simulink model "Lista4"  (R2023a)
settings: Solver=VariableStepAuto  StartTime=0.0  StopTime=10.0  RelTol=1e-3
libraries: fl_lib x8, nesl_utility x3
settings Model: Creator=gutoc  LastModifiedBy=gutoc

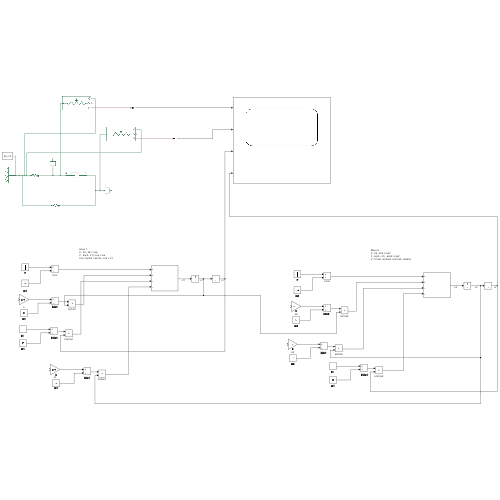
[thumbnail: Simulink's stored preview of the top-level diagram]
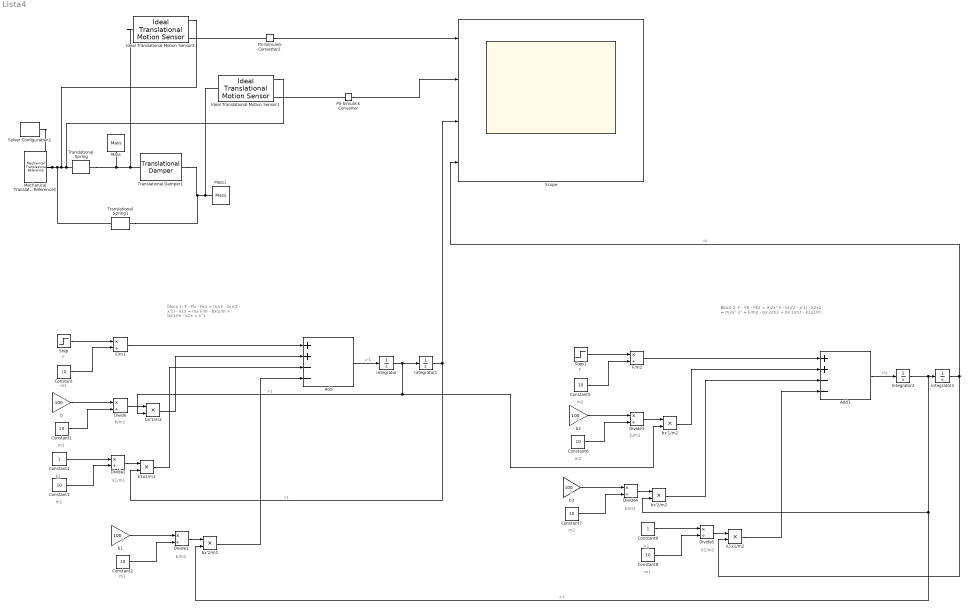
== system Lista4 ==
  note: Bloco 2:
      | F - Fb - Fk2 = m2x''
      | F - b(x'2 - x'1) - k2x2 = m2x"
      | x" = F/m2 - bx'2/m2 + bx'1/m2 - k2x2/m
  note: b
  note: m2
  note: b/m1
  note: m1
  note: k1
  note: m2
  note: k1/m1
  note: b/m2
  note: F
  note: m2
  note: b
  note: b
  note: bloco 1:
      | F - Fb - Fk1 = ma
      | F - b(x'2 - x'1) - k1x = ma
      | F/m - bx'2/m + bx'1/m - k1x = x"1
  note: m1
  note: m1
  note: b/m1
  note: m1
  note: k1
  note: m1
  note: k1/m1
  note: b/m1
  note: F
  Add : Sum  Inputs=++--
  Add1 : Sum  Inputs=++--
  Constant{,1..3,5..8} (8 alike) : Constant  Value=10
  Constant4 : Constant
  Constant9 : Constant
  Divide{,1..5} (6 alike) : Product  Inputs=*/
  F/m1 : Product  Inputs=*/
  F/m2 : Product  Inputs=*/
  Ideal Translational Motion Sensor1 : fl_lib/Mechanical/Mechanical Sensors/Ideal Translational Motion Sensor  reference=foundation.enum.MeasurementReference.difference  acceleration_port=false  velocity_port=true  position_port=true  offset=0 m
  Ideal Translational Motion Sensor3 : fl_lib/Mechanical/Mechanical Sensors/Ideal Translational Motion Sensor  reference=foundation.enum.MeasurementReference.difference  acceleration_port=false  velocity_port=true  position_port=true  offset=0 m
  Integrator{,1..3} (4 alike) : Integrator
  Mass : fl_lib/Mechanical/Translational Elements/Mass  mass=1 kg  num_ports=foundation.enum.numPorts2.one  v_specify=off  v_priority=High  v=0 m/s  v_nominal_specify=off  v_nominal_unit=m/s  v_nominal_value=1  f_specify=off  f_priority=None  f=0 N  f_nominal_specify=off  f_nominal_unit=N  f_nominal_value=1
  Mass1 : fl_lib/Mechanical/Translational Elements/Mass  mass=2 kg  num_ports=foundation.enum.numPorts2.one  v_specify=off  v_priority=High  v=0 m/s  v_nominal_specify=off  v_nominal_unit=m/s  v_nominal_value=1  f_specify=off  f_priority=None  f=0 N  f_nominal_specify=off  f_nominal_unit=N  f_nominal_value=1
  Mechanical Translational Reference1 : fl_lib/Mechanical/Translational Elements/Mechanical Translational Reference
  PS-Simulink Converter : nesl_utility/PS-Simulink Converter  PhysicalDomain=network_engine_domain  SubClassName=ps_output  LeftPortType=input  RightPortType=output  PseudoPeriodic=off  Frequencies=[]  VectorFormat=inherit  Unit=inherit  AffineConversion=off
  PS-Simulink Converter2 : nesl_utility/PS-Simulink Converter  PhysicalDomain=network_engine_domain  SubClassName=ps_output  LeftPortType=input  RightPortType=output  PseudoPeriodic=off  Frequencies=[]  VectorFormat=inherit  Unit=inherit  AffineConversion=off
  Scope : Scope  NumInputPorts=4
  Solver Configuration1 : nesl_utility/Solver Configuration  PhysicalDomain=network_engine_domain  SubClassName=solver  LeftPortType=input  RightPortType=generic  Tones=[]  Harmonics=[]  SimulateNoise=off  Profile=off  UseLocalSampling=off  EnableSwitchedLinearOptims=on  FrequencyDomain=off  UseCCode=off  RelTol=0.001  AbsTol=1e-06  MinStep=1e-09  ToWorkspace=off  RevertToSquareIcSolve=off  NumHomotopyIterations=100  PhasorMode=off  PhasorModeNumHarmonics=1  ConsistencySolver=NEWTON_FTOL  IndexReductionMethod=DerivativeReplacement  DoDC=off  ResidualTolerance=1e-09  ConsistencyTolSource=GLOBAL  ConsistencyAbsTol=0.001  ConsistencyRelTol=0.001  ConsistencyTolFactor=0.001  UseLocalSolver=off  LocalSolverChoice=NE_BACKWARD_EULER_ADVANCER  ResolveIndetEquations=on  FunctionEvalNumThread=1  LocalSolverSampleTime=0.001  DoFixedCost=off  MaxNonlinIter=3  MaxModeIter=2  ComputeImpulses=off  ImpulseIterations=2  LinearAlgebra=Sparse  LinearAlgebraNumThread=0  EquationFormulation=NE_TIME_EF  DelaysMemoryBudget=1024  AutomaticFiltering=on  FilteringTimeConstant=0.001  PartitionStorageMethod=AS_NEEDED  PartitionMemoryBudget=1024  PartitionMethod=FAST
  Step : Step  SampleTime=0
  Step1 : Step  SampleTime=0
  Translational Damper1 : fl_lib/Mechanical/Translational Elements/Translational Damper  D=100 N/(m/s)  v_specify=off  v_priority=None  v=0 m/s  v_nominal_specify=off  v_nominal_unit=m/s  v_nominal_value=1  f_specify=off  f_priority=None  f=0 N  f_nominal_specify=off  f_nominal_unit=N  f_nominal_value=1
  Translational Spring : fl_lib/Mechanical/Translational Elements/Translational Spring  spr_rate=1000 N/m  v_specify=off  v_priority=None  v=0 m/s  v_nominal_specify=off  v_nominal_unit=m/s  v_nominal_value=1  f_specify=off  f_priority=None  f=0 N  f_nominal_specify=off  f_nominal_unit=N  f_nominal_value=1  x_specify=off  x_priority=High  x=0 m  x_nominal_specify=off  x_nominal_unit=m  x_nominal_value=1
  Translational Spring1 : fl_lib/Mechanical/Translational Elements/Translational Spring  spr_rate=1000 N/m  v_specify=off  v_priority=None  v=0 m/s  v_nominal_specify=off  v_nominal_unit=m/s  v_nominal_value=1  f_specify=off  f_priority=None  f=0 N  f_nominal_specify=off  f_nominal_unit=N  f_nominal_value=1  x_specify=off  x_priority=High  x=0 m  x_nominal_specify=off  x_nominal_unit=m  x_nominal_value=1
  b{,1..3} (4 alike) : Gain  Gain=100
  bx'1/m1 : Product
  bx'1/m2 : Product
  bx'2/m1 : Product
  bx'2/m2 : Product
  k1x1/m1 : Product
  k1x1/m2 : Product
  wires:
  PS-Simulink Converter/1 -> Scope/2
  PS-Simulink Converter2/1 -> Scope/1
  bx'2/m2/1 -> Add1/3
  F/m2/1 -> Add1/1
  Step1/1 -> F/m2/1
  Divide4/1 -> bx'2/m2/1
  b3/1 -> Divide4/1
  Constant7/1 -> Divide4/2
  Divide3/1 -> bx'1/m2/1
  Constant9/1 -> Divide5/1
  Constant6/1 -> Divide3/2
  Divide5/1 -> k1x1/m2/1
  Constant8/1 -> Divide5/2
  Integrator2/1 -> bx'2/m1/2, bx'2/m2/2, Integrator3/1  "x'2"
  Constant5/1 -> F/m2/2
  Integrator3/1 -> Scope/4, k1x1/m2/2  "x2"
  k1x1/m2/1 -> Add1/4
  Add1/1 -> Integrator2/1  "x\"2"
  bx'1/m2/1 -> Add1/2
  b2/1 -> Divide3/1
  F/m1/1 -> Add/1
  Step/1 -> F/m1/1
  Divide1/1 -> bx'2/m1/1
  b1/1 -> Divide1/1
  Constant2/1 -> Divide1/2
  Divide/1 -> bx'1/m1/1
  Constant4/1 -> Divide2/1
  b/1 -> Divide/1
  Constant1/1 -> Divide/2
  Divide2/1 -> k1x1/m1/1
  Constant3/1 -> Divide2/2
  Integrator/1 -> bx'1/m2/2, bx'1/m1/2, Integrator1/1  "x'1"
  Constant/1 -> F/m1/2
  Integrator1/1 -> Scope/3, k1x1/m1/2  "x1"
  k1x1/m1/1 -> Add/3
  Add/1 -> Integrator/1  "x\"1"
  bx'1/m1/1 -> Add/2
  bx'2/m1/1 -> Add/4
  connections:
  Translational Spring/RConn1 -- Ideal Translational Motion Sensor1/RConn1 -- Ideal Translational Motion Sensor3/RConn1 -- Translational Spring1/RConn1 -- Solver Configuration1/RConn1 -- Mechanical Translational Reference1/LConn1
  Translational Spring/LConn1 -- Ideal Translational Motion Sensor3/LConn1 -- Translational Damper1/LConn1 -- Mass/LConn1
  Translational Damper1/RConn1 -- Translational Spring1/LConn1 -- Ideal Translational Motion Sensor1/LConn1 -- Mass1/LConn1
  Ideal Translational Motion Sensor1/RConn3 -- PS-Simulink Converter/LConn1
  Ideal Translational Motion Sensor3/RConn3 -- PS-Simulink Converter2/LConn1
